simulink model "sampleModel213"  (R2021b)
settings: Solver=VariableStepAuto  StartTime=0.0  StopTime=10.0  RelTol=1e-3
undefined symbols (not defined in the file or in its folder): DiscIntNeverNeededParam
libraries: simulink x6
settings Model: Creator=user  LastModifiedBy=user

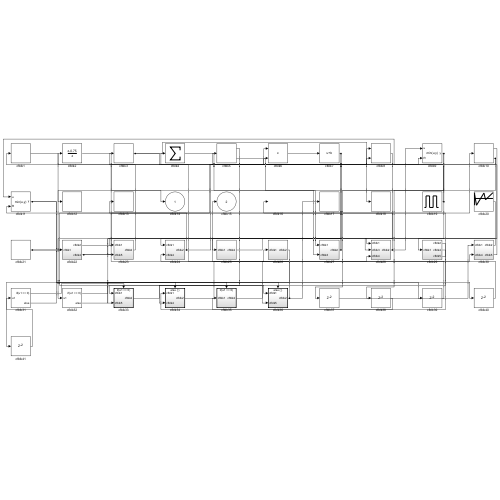
[thumbnail: Simulink's stored preview of the top-level diagram]
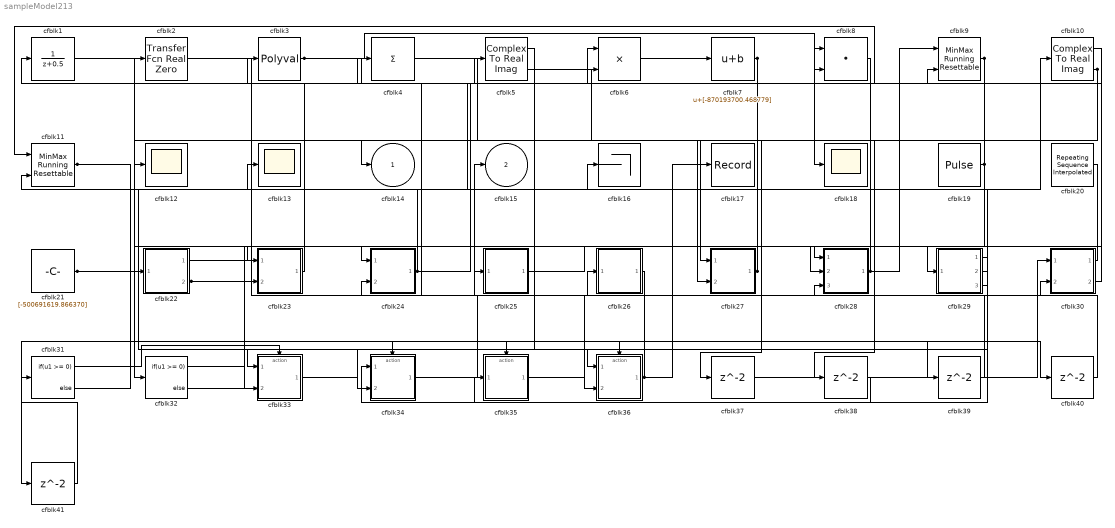
== system sampleModel213 ==
  cfblk1 : DiscreteTransferFcn  SampleTime=1
  cfblk10 : ComplexToRealImag
  cfblk11 : simulink/Math Operations/MinMax Running Resettable  Function=min  vinit=0.0
  cfblk12 : Scope
  cfblk13 : Scope
  cfblk16 : Terminator
  cfblk17 : Record  FileSettingsInternal="{\"entries\":[{\"content\":{\"excelSettings\":{\"content\":{},\"type\":\"Streamout.ExcelSettings\"}},\"type\":\"Streamout.FileSettingStorage\",\"uuid\":\"28e4c51c-1937-41a0-a133-1cff96515ed7\"}],\"packageUris\":[\"http://schema.mathworks.com/mf0/streamout_blocks/R2020a\"],\"version\":\"1.0\"}"  SignalsInternal="{\"entries\":[{\"content\":{\"signals\":[{\"content\":{\"blockPath\":[\"sampleModel213/cfblk17\"],\"channel\":[],\"dimensions\":[1],\"domain\":\"sampleModel213/cfblk17\",\"lineColor\":\"#64d413\",\"plots\":[1],\"port\":1,\"sid\":[\"\"],\"signalID\":8292,\"signalName\":\"cfblk36\"},\"type\":\"RecordBlkView.Signal\",\"uuid\":\"0845694e-0171-4560-bc0c-7199e26a6a20\"}]},\"type\":\"RecordBlkView.InputSignals\",\"uuid\":\"2b9fda15-a465-4095-a7b0-130934ec02d6\"}],\"packageUris\":[\"http://schema.mathworks.com/mf0/streamout_blocks/R2020a\"],\"version\":\"1.0\"}"  VisualizationBindings="{\"sparklinesplugin\":{\"info\":[{\"bindingParametersList\":[],\"subplotID\":1}]}}"
  cfblk18 : Scope
  cfblk19 : DiscretePulseGenerator  PulseType=Time based  Amplitude=[357934836.344518]  Period=[18432357.661940]  PulseWidth=5  PhaseDelay=[3.000000]
  cfblk2 : simulink/Discrete/Transfer Fcn Real Zero  ZeroZ=0.75  ICPrevInput=0.0  DoSatur=off
      settings: SourceProductBaseCode=SL
  cfblk20 : simulink/Sources/Repeating Sequence Interpolated  OutValues=[517191139.030052, -869290179.634214, 713681820.510494, -174885215.341994, 787108902.739112]  TimeValues=[0 0.1 0.5 0.6 1].'  LookUpMeth=Interpolation-Use End Values  tsamp=0.01  OutMin=[]  OutMax=[]  OutDataTypeStr=double  OutputDataTypeScalingMode=double  OutDataType=fixdt(0,8)  OutScaling=2^-10
  cfblk21 : Constant  Value=[-500691619.866370]  SampleTime=1
  cfblk22 : Subsystem
  cfblk23 : Subsystem
  cfblk24 : Subsystem
  cfblk25 : Subsystem
  cfblk26 : Subsystem
  cfblk27 : Subsystem
  cfblk28 : Subsystem
  cfblk29 : Subsystem
  cfblk3 : Polyval  Coefs=[ +2.081618890e-019, -1.441693666e-014, +4.719686976e-010, -8.536869453e-006, +1.621573104e-001, -8.087801117e+001 ]
  cfblk30 : Subsystem
  cfblk31 : If  IfExpression=u1 >= 0  SampleTime=1
  cfblk32 : If  IfExpression=u1 >= 0  SampleTime=1
  cfblk33 : Subsystem  TreatAsAtomicUnit=on
  cfblk34 : Subsystem  TreatAsAtomicUnit=on
  cfblk35 : Subsystem  TreatAsAtomicUnit=on
  cfblk36 : Subsystem  TreatAsAtomicUnit=on
  cfblk{37..41} (5 alike) : Delay  SampleTime=1
  cfblk4 : Sum  Inputs=+
  cfblk5 : ComplexToRealImag
  cfblk6 : Product
  cfblk7 : Bias  Bias=[-870193700.468779]
  cfblk8 : DotProduct  InputSameDT=on  OutDataTypeStr=Inherit: Inherit via internal rule
  cfblk9 : simulink/Math Operations/MinMax Running Resettable  Function=min  vinit=0.0
  cfblk14 : Outport
  cfblk15 : Outport  Port=2
  wires:
  cfblk7/1 -> cfblk24/1(cfblk1), cfblk33/2(cfblk5)
  cfblk2/1 -> cfblk14/1
  cfblk29/1(cfblk2) -> cfblk34/1(cfblk1)
  cfblk36/1(cfblk2) -> cfblk15/1, cfblk17/1
  cfblk34/1(cfblk2) -> cfblk26/1(cfblk1)
  cfblk8/1 -> cfblk25/1(cfblk1)
  cfblk25/1(cfblk2) -> cfblk28/1(cfblk1)
  cfblk28/1(cfblk2) -> cfblk16/1, cfblk9/1
  cfblk3/1 -> cfblk18/1, cfblk8/2
  cfblk22/1(cfblk2) -> cfblk6/1
  cfblk27/1(cfblk2) -> cfblk1/1, cfblk22/1(cfblk1)
  cfblk33/1(cfblk2) -> cfblk36/1(cfblk1)
  cfblk1/1 -> cfblk32/1
  cfblk10/1 -> cfblk29/1(cfblk1)
  cfblk23/1(cfblk2) -> cfblk3/1
  cfblk22/2(cfblk4) -> cfblk8/1, cfblk28/3(cfblk4)
  cfblk9/1 -> cfblk37/1, cfblk38/1
  cfblk19/1 -> cfblk11/1, cfblk23/2(cfblk5), cfblk6/2
  cfblk10/2 -> cfblk12/1, cfblk5/1
  cfblk6/1 -> cfblk7/1
  cfblk35/1(cfblk2) -> cfblk30/2(cfblk4)
  cfblk4/1 -> cfblk27/1(cfblk1)
  cfblk29/2(cfblk4) -> cfblk33/1(cfblk1)
  cfblk5/1 -> cfblk34/2(cfblk4)
  cfblk21/1 -> cfblk10/1, cfblk36/2(cfblk5)
  cfblk30/1(cfblk2) -> cfblk28/2(cfblk3)
  cfblk24/1(cfblk2) -> cfblk11/2, cfblk9/2
  cfblk30/2(cfblk5) -> cfblk2/1
  cfblk20/1 -> cfblk23/1(cfblk1)
  cfblk5/2 -> cfblk27/2(cfblk3)
  cfblk29/3(cfblk5) -> cfblk13/1
  cfblk11/1 -> cfblk39/1, cfblk40/1
  cfblk31/1 -> cfblk33/Action
  cfblk31/2 -> cfblk34/Action
  cfblk32/1 -> cfblk35/Action
  cfblk32/2 -> cfblk36/Action
  cfblk37/1 -> cfblk30/1(cfblk1)
  cfblk38/1 -> cfblk35/1(cfblk1)
  cfblk39/1 -> cfblk4/1
  cfblk40/1 -> cfblk24/2(cfblk4)
  cfblk26/1(cfblk2) -> cfblk41/1
  cfblk41/1 -> cfblk31/1

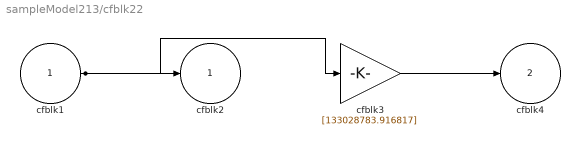
== system sampleModel213/cfblk22 ==
  cfblk1 : Inport
  cfblk3 : Gain  Gain=[133028783.916817]
  cfblk2 : Outport
  cfblk4 : Outport  Port=2
  wires:
  cfblk1/1 -> cfblk2/1, cfblk3/1
  cfblk3/1 -> cfblk4/1

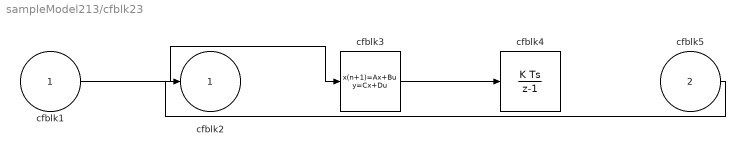
== system sampleModel213/cfblk23 ==
  cfblk1 : Inport
  cfblk5 : Inport  Port=2
  cfblk3 : DiscreteStateSpace
  cfblk4 : DiscreteIntegrator  ICPrevOutput=DiscIntNeverNeededParam  ICPrevScaledInput=DiscIntNeverNeededParam
  cfblk2 : Outport
  wires:
  cfblk3/1 -> cfblk4/1
  cfblk1/1 -> cfblk3/1
  cfblk5/1 -> cfblk2/1

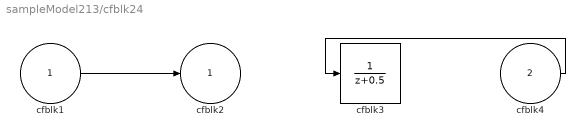
== system sampleModel213/cfblk24 ==
  cfblk1 : Inport
  cfblk4 : Inport  Port=2
  cfblk3 : DiscreteTransferFcn  SampleTime=1
  cfblk2 : Outport
  wires:
  cfblk1/1 -> cfblk2/1
  cfblk4/1 -> cfblk3/1

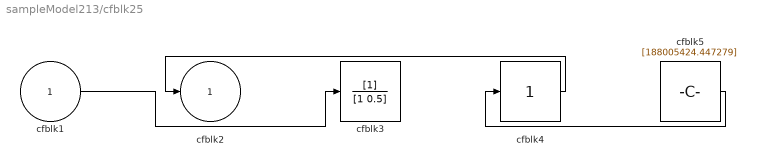
== system sampleModel213/cfblk25 ==
  cfblk1 : Inport
  cfblk3 : DiscreteFilter  SampleTime=1
  cfblk4 : simulink/Math Operations/Slider Gain  gain=1  low=0  high=2
  cfblk5 : Constant  Value=[188005424.447279]  SampleTime=1
  cfblk2 : Outport
  wires:
  cfblk4/1 -> cfblk2/1
  cfblk1/1 -> cfblk3/1
  cfblk5/1 -> cfblk4/1

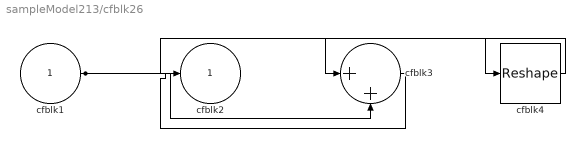
== system sampleModel213/cfblk26 ==
  cfblk1 : Inport
  cfblk3 : Sum  Inputs=|++
  cfblk4 : Reshape
  cfblk2 : Outport
  wires:
  cfblk4/1 -> cfblk3/1
  cfblk1/1 -> cfblk3/2, cfblk4/1
  cfblk3/1 -> cfblk2/1

== system sampleModel213/cfblk27 ==
  cfblk1 : Inport
  cfblk3 : Inport  Port=2
  cfblk2 : Outport
  wires:
  cfblk1/1 -> cfblk2/1

== system sampleModel213/cfblk28 ==
  cfblk1 : Inport
  cfblk3 : Inport  Port=2
  cfblk4 : Inport  Port=3
  cfblk2 : Outport
  wires:
  cfblk1/1 -> cfblk2/1

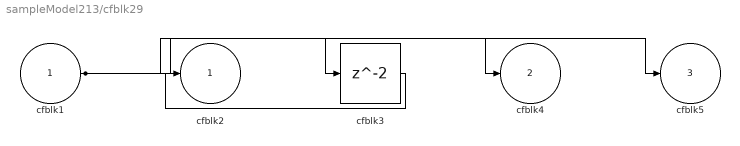
== system sampleModel213/cfblk29 ==
  cfblk1 : Inport
  cfblk3 : Delay  SampleTime=1
  cfblk2 : Outport
  cfblk4 : Outport  Port=2
  cfblk5 : Outport  Port=3
  wires:
  cfblk1/1 -> cfblk5/1, cfblk4/1, cfblk3/1
  cfblk3/1 -> cfblk2/1

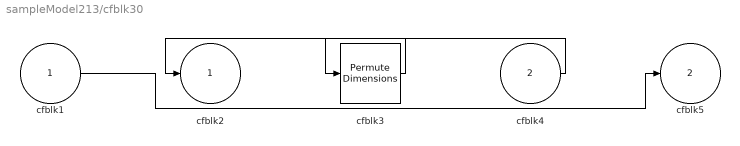
== system sampleModel213/cfblk30 ==
  cfblk1 : Inport
  cfblk4 : Inport  Port=2
  cfblk3 : PermuteDimensions
  cfblk2 : Outport
  cfblk5 : Outport  Port=2
  wires:
  cfblk3/1 -> cfblk2/1
  cfblk1/1 -> cfblk5/1
  cfblk4/1 -> cfblk3/1

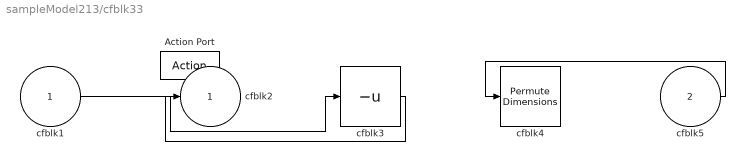
== system sampleModel213/cfblk33 ==
  cfblk1 : Inport
  cfblk5 : Inport  Port=2
  Action Port : ActionPort  ActionPortLabel=if(u1 >= 0)
  cfblk3 : UnaryMinus
  cfblk4 : PermuteDimensions
  cfblk2 : Outport
  wires:
  cfblk5/1 -> cfblk4/1
  cfblk1/1 -> cfblk3/1
  cfblk3/1 -> cfblk2/1

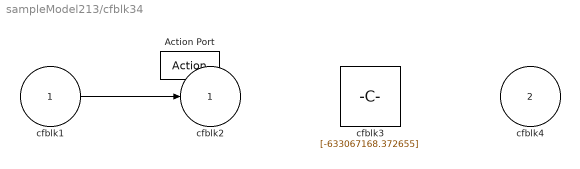
== system sampleModel213/cfblk34 ==
  cfblk1 : Inport
  cfblk4 : Inport  Port=2
  Action Port : ActionPort  ActionPortLabel=else
  cfblk3 : Constant  Value=[-633067168.372655]  SampleTime=1
  cfblk2 : Outport
  wires:
  cfblk1/1 -> cfblk2/1

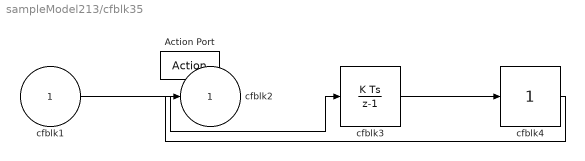
== system sampleModel213/cfblk35 ==
  cfblk1 : Inport
  Action Port : ActionPort  ActionPortLabel=if(u1 >= 0)
  cfblk3 : DiscreteIntegrator  SampleTime=-1  ICPrevOutput=DiscIntNeverNeededParam  ICPrevScaledInput=DiscIntNeverNeededParam
  cfblk4 : simulink/Math Operations/Slider Gain  gain=1  low=0  high=2
  cfblk2 : Outport
  wires:
  cfblk1/1 -> cfblk3/1
  cfblk3/1 -> cfblk4/1
  cfblk4/1 -> cfblk2/1

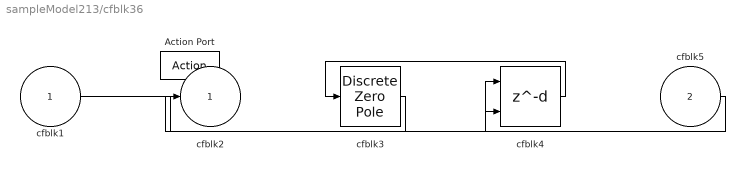
== system sampleModel213/cfblk36 ==
  cfblk1 : Inport
  cfblk5 : Inport  Port=2
  Action Port : ActionPort  ActionPortLabel=else
  cfblk3 : DiscreteZeroPole  Poles=[0 0.5]  Gain=1  SampleTime=-1
  cfblk4 : Delay  DelayLengthSource=Input port
      settings: InputPortMap=u0,p1
  cfblk2 : Outport
  wires:
  cfblk4/1 -> cfblk3/1
  cfblk5/1 -> cfblk4/1
  cfblk1/1 -> cfblk4/2
  cfblk3/1 -> cfblk2/1
